simulink model "mod3_CRFF_cct_1bit"  (R2013a)
settings: Solver=FixedStepDiscrete  StartTime=0.0  StopTime=80e-3  RelTol=1e-3
undefined symbols (not defined in the file): Fs, modctrl
libraries: dspsigops x3, dspsrcs4 x1
settings Model: Creator=amyles  LastModifiedBy=amyles
settings DataIOCC: LimitDataPoints=off  MaxDataPoints=50000  SignalLoggingSaveFormat=ModelDataLogs
settings OptimizationCC: InlineParams=on  ExpressionDepthLimit=2147483647
settings DebuggingCC: FcnCallInpInsideContextMsg=UseLocalSettings  StrictBusMsg=Warning
settings ModelReferenceCC: ModelReferenceNumInstancesAllowed=Single
settings GRTTargetCC: CombineOutputUpdateFcns=off  GRTInterface=on

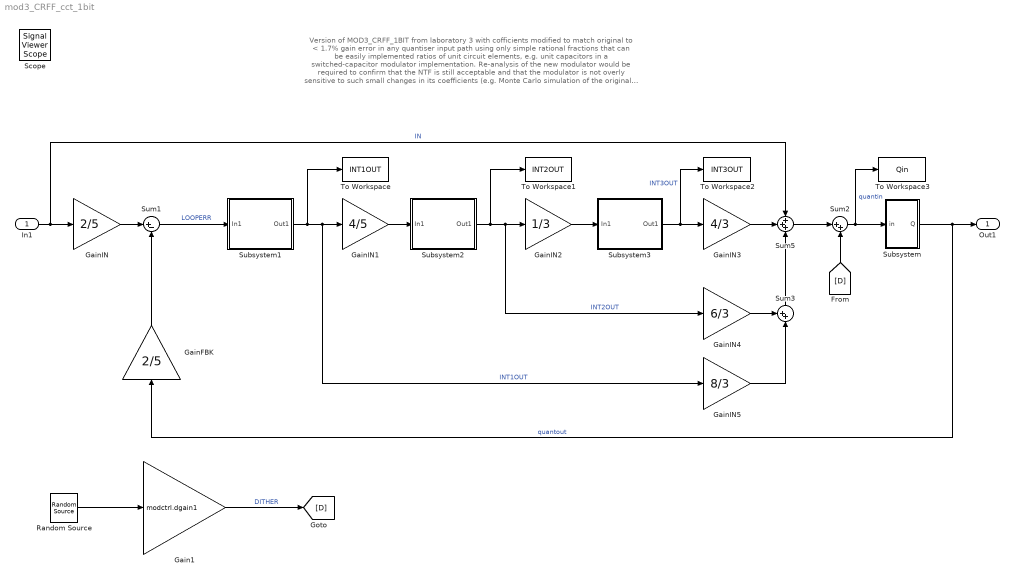
== system mod3_CRFF_cct_1bit ==
  note: Version of MOD3_CRFF_1BIT from laboratory 3 with cofficients modified to match original to < 1.7% gain error in any quantiser
      | input path using only simple rational fractions that can be easily implemented ratios of unit circuit elements, e.g. unit capacitors
      | in a switched-capacitor modulator implementation. Re-analysis of the new modulator would be required to confirm that
      | the NTF is still acceptable and that the modulator is not overly sensitive to such small changes in its coefficients (e.g. Monte
      | Carlo simulation of the original modulator). Alarm bells should ring if you do find your modulator to be highly sensitive to small
      | variations in it's coefficients - such as seen with the error-feedback implementation from laboratory 2 or some MASH types - because
      | in reality for all analogue modulators (ADCs) there WILL be unavoidable small variations due to manufacturing variability.
  In1 : Inport
  Gain1 : Gain  Gain=modctrl.dgain1
      settings: AttributesFormatString=Dither level adjust
  GainFBK : Gain  Gain=2/5
  GainIN : Gain  Gain=2/5
  GainIN1 : Gain  Gain=4/5
  GainIN2 : Gain  Gain=1/3
  GainIN3 : Gain  Gain=4/3
  GainIN4 : Gain  Gain=6/3
  GainIN5 : Gain  Gain=8/3
  Random Source : dspsrcs4/Random Source  SrcType=Uniform  NormMethod=Ziggurat  CltLength=12  MinVal=-1  MaxVal=1  MeanVal=0  VarVal=1  RepMode=Not repeatable  rawSeed=1  IsInherit=off  SampMode=Discrete  SampTime=1/Fs  SampFrame=1  DataType=Double  OutComplex=Real
      settings: AttributesFormatString=Dither source
  Subsystem : Subsystem
      settings: AttributesFormatString=1-bit quantiser
  Subsystem1 : Subsystem
      settings: AttributesFormatString=Leaky delaying integrator
  Subsystem2 : Subsystem
      settings: AttributesFormatString=Leaky DELAYLESS integrator
  Subsystem3 : Subsystem
      settings: AttributesFormatString=Leaky delaying integrator
  Sum1 : Sum  Inputs=|+-
      settings: AttributesFormatString=Modulator input\nloop servo error (input - fbk)
  Sum2 : Sum  Inputs=|++
  Sum3 : Sum  Inputs=++|
  Sum5 : Sum  Inputs=+++
  To Workspace : ToWorkspace  VariableName=INT1OUT  SampleTime=-1
  To Workspace1 : ToWorkspace  VariableName=INT2OUT  SampleTime=-1
  To Workspace2 : ToWorkspace  VariableName=INT3OUT  SampleTime=-1
  To Workspace3 : ToWorkspace  VariableName=Qin  SampleTime=-1
  Out1 : Outport
  Scope : SignalViewerScope  IOType=viewer  NumInputPorts=4  ZoomMode=yonly  RefreshTime=0.035000
      settings: ShowLegends=on  YMin=-5~-5~-5~-5  YMax=5~5~5~5
  wires:
  Sum1/1 -> Subsystem1/1(In1)  "LOOPERR"
  In1/1 -> GainIN/1, Sum5/1  "IN"
  Sum2/1 -> Subsystem/1(in), To Workspace3/1  "quantin"
  Subsystem/1(Q) -> Out1/1, GainFBK/1  "quantout"
  Random Source/1 -> Gain1/1
  Subsystem1/1(Out1) -> GainIN1/1, GainIN5/1, To Workspace/1  "INT1OUT"
  GainIN1/1 -> Subsystem2/1(In1)
  Subsystem2/1(Out1) -> GainIN2/1, GainIN4/1, To Workspace1/1  "INT2OUT"
  Gain1/1 -> [D]  "DITHER"
  GainFBK/1 -> Sum1/2
  GainIN/1 -> Sum1/1
  Subsystem3/1(Out1) -> GainIN3/1, To Workspace2/1  "INT3OUT"
  Sum5/1 -> Sum2/1
  [D] -> Sum2/2
  GainIN2/1 -> Subsystem3/1(In1)
  GainIN3/1 -> Sum5/2
  GainIN4/1 -> Sum3/1
  Sum3/1 -> Sum5/3
  GainIN5/1 -> Sum3/2

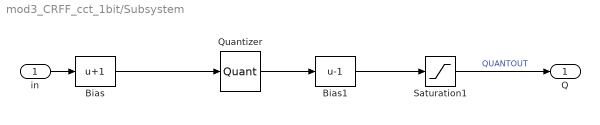
== system mod3_CRFF_cct_1bit/Subsystem ==
  in : Inport
  Bias : Bias  Bias=1
      settings: AttributesFormatString=Need offset to give\nMID-RISE quantiser
  Bias1 : Bias  Bias=-1
  Quantizer : Quantizer  QuantizationInterval=2  LinearizeAsGain=off
  Saturation1 : Saturate  UpperLimit=1  LowerLimit=-1
      settings: AttributesFormatString=Limit quantiser\noutput to +/-1
  Q : Outport
  wires:
  Bias/1 -> Quantizer/1
  Quantizer/1 -> Bias1/1
  Bias1/1 -> Saturation1/1
  in/1 -> Bias/1
  Saturation1/1 -> Q/1  "QUANTOUT"

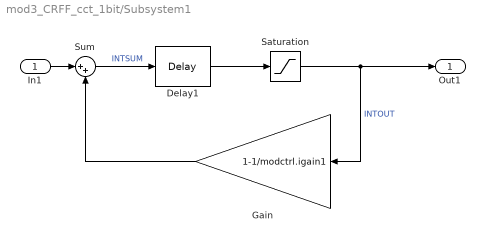
== system mod3_CRFF_cct_1bit/Subsystem1 ==
  In1 : Inport
  Delay1 : dspsigops/Delay  InputProcessing=Inherited (this choice will be removed - see release notes)  dly_unit=Samples  delay=1  ic_detail=off  dif_ic_for_ch=off  dif_ic_for_dly=off  ic=0  reset_popup=None
  Gain : Gain  Gain=1-1/modctrl.igain1
      settings: AttributesFormatString=Integrator leakage
  Saturation : Saturate  UpperLimit=modctrl.isat1  LowerLimit=-(modctrl.isat1)
  Sum : Sum  Inputs=|++
      settings: AttributesFormatString=Integrator summer
  Out1 : Outport
  wires:
  Sum/1 -> Delay1/1  "INTSUM"
  Gain/1 -> Sum/2
  Saturation/1 -> Gain/1, Out1/1  "INTOUT"
  In1/1 -> Sum/1
  Delay1/1 -> Saturation/1

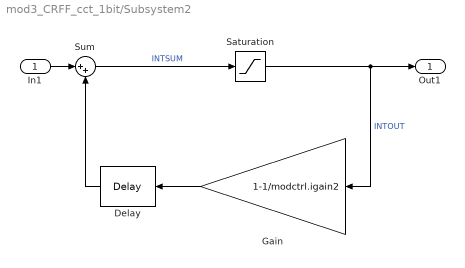
== system mod3_CRFF_cct_1bit/Subsystem2 ==
  In1 : Inport
  Delay : dspsigops/Delay  InputProcessing=Inherited (this choice will be removed - see release notes)  dly_unit=Samples  delay=1  ic_detail=off  dif_ic_for_ch=off  dif_ic_for_dly=off  ic=0  reset_popup=None
  Gain : Gain  Gain=1-1/modctrl.igain2
      settings: AttributesFormatString=Integrator leakage
  Saturation : Saturate  UpperLimit=modctrl.isat2  LowerLimit=-(modctrl.isat2)
  Sum : Sum  Inputs=|++
      settings: AttributesFormatString=Integrator summer
  Out1 : Outport
  wires:
  In1/1 -> Sum/1
  Saturation/1 -> Out1/1, Gain/1  "INTOUT"
  Gain/1 -> Delay/1
  Sum/1 -> Saturation/1  "INTSUM"
  Delay/1 -> Sum/2

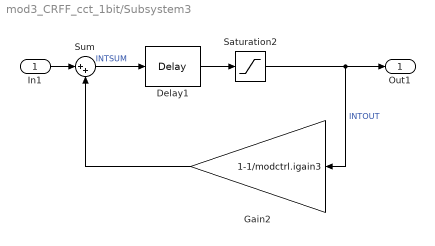
== system mod3_CRFF_cct_1bit/Subsystem3 ==
  In1 : Inport
  Delay1 : dspsigops/Delay  InputProcessing=Inherited (this choice will be removed - see release notes)  dly_unit=Samples  delay=1  ic_detail=off  dif_ic_for_ch=off  dif_ic_for_dly=off  ic=0  reset_popup=None
  Gain2 : Gain  Gain=1-1/modctrl.igain3
      settings: AttributesFormatString=Integrator leakage
  Saturation2 : Saturate  UpperLimit=modctrl.isat3  LowerLimit=-(modctrl.isat3)
  Sum : Sum  Inputs=|++
      settings: AttributesFormatString=Integrator summer
  Out1 : Outport
  wires:
  Sum/1 -> Delay1/1  "INTSUM"
  Gain2/1 -> Sum/2
  Saturation2/1 -> Gain2/1, Out1/1  "INTOUT"
  In1/1 -> Sum/1
  Delay1/1 -> Saturation2/1
